simulink model "A1_cc_R2017b"  (R2020b)
settings: Solver=ode45  StartTime=0.0  StopTime=100  MaxStep=1e-3  RelTol=1e-3
values from neighbouring files (symbols this model uses):
  a = data(2)    [A1_10.m]    (also in problem6.m = 270)
  b = data(3)    [A1_10.m]    (also in problem6.m = 11000)
  g = 9.82    [A1_10.m]
  Ki = 0.0    (= 0)    [A1_10.m]
  Kp = 0.0    (= 0)    [A1_10.m]
settings Model: Creator=jofr  LastModifiedBy=jofr
settings DataIOCC: LimitDataPoints=on  SaveFormat=Array  SignalLoggingSaveFormat=ModelDataLogs  ReturnWorkspaceOutputs=off
settings OptimizationCC: BlockReduction=off  BooleanDataType=off  LifeSpan=inf
settings DebuggingCC: SaveWithParameterizedLinksMsg=none  UnderspecifiedInitializationDetection=Classic  MergeDetectMultiDrivingBlocksExec=none  SignalResolutionControl=TryResolveAllWithWarning  MultiTaskDSMMsg=warning  MultiTaskCondExecSysMsg=none  SFUnexpectedBacktrackingDiag=warning  SFNoUnconditionalDefaultTransitionDiag=warning  SFExecutionAtInitializationDiag=none  ArithmeticOperatorsInVariantConditions=warning
settings HardwareCC: ProdBitPerPointer=32  ProdBitPerSizeT=32  ProdBitPerPtrDiffT=32  ProdLargestAtomicFloat=None  ProdIntDivRoundTo=Undefined  ProdEndianess=Unspecified  ProdWordSize=32  ProdHWDeviceType=32-bit Generic  TargetUnknown=on
settings ModelReferenceCC: PropagateSignalLabelsOutOfModel=off
settings SFSimCC: SimUseLocalCustomCode=off  CustomCodeUndefinedFunction=UseInterfaceOnly
settings RTWCC: RTWUseLocalCustomCode=off
settings CodeAppCC: StateflowObjectComments=on
settings GRTTargetCC: TargetLangStandard=C89/C90 (ANSI)
settings ConfigComp: CovMetricSettings=dw  CovSaveCumulativeToWorkspaceVar=on  CovSaveSingleToWorkspaceVar=on  CovExternalEMLEnable=off

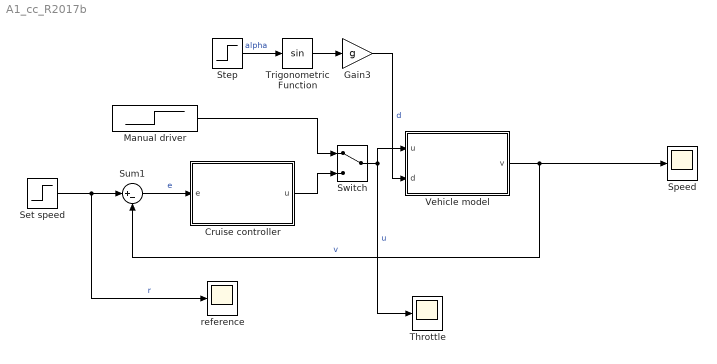
== system A1_cc_R2017b ==
  Cruise controller : Subsystem
  Gain3 : Gain  Gain=g
  Manual driver : Step  Before=25*a/b  After=30*a/b  SampleTime=0
  Set speed : Step  Before=25  After=30  SampleTime=0
  Speed : Scope
  Step : Step  Time=1000  After=0.1  SampleTime=0
  Sum1 : Sum  Inputs=|+-
  Switch : ManualSwitch
  Throttle : Scope
  Trigonometric Function : Trigonometry
  Vehicle model : Subsystem
  reference : Scope
  wires:
  Trigonometric Function/1 -> Gain3/1
  Step/1 -> Trigonometric Function/1  "alpha"
  Set speed/1 -> Sum1/1, reference/1  "r"
  Sum1/1 -> Cruise controller/1(e)  "e"
  Vehicle model/1(v) -> Sum1/2, Speed/1  "v"
  Gain3/1 -> Vehicle model/2(d)  "d"
  Switch/1 -> Throttle/1, Vehicle model/1(u)  "u"
  Cruise controller/1(u) -> Switch/2
  Manual driver/1 -> Switch/1

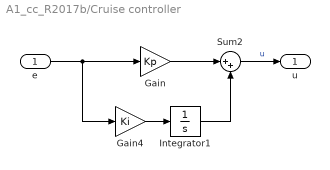
== system A1_cc_R2017b/Cruise controller ==
  e : Inport
  Gain : Gain  Gain=Kp
  Gain4 : Gain  Gain=Ki
  Integrator1 : Integrator  InitialCondition=a*25/b
  Sum2 : Sum  Inputs=|++
  u : Outport
  wires:
  Gain4/1 -> Integrator1/1
  Gain/1 -> Sum2/1
  Sum2/1 -> u/1  "u"
  Integrator1/1 -> Sum2/2
  e/1 -> Gain4/1, Gain/1

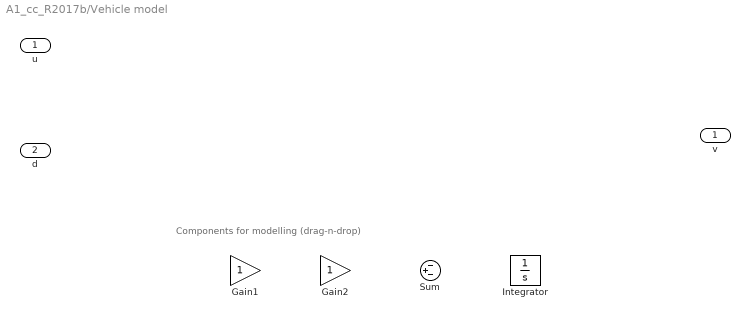
== system A1_cc_R2017b/Vehicle model ==
  note: Components for modelling (drag-n-drop)
  u : Inport
  d : Inport  Port=2
  Gain1 : Gain
  Gain2 : Gain
  Integrator : Integrator  InitialCondition=25
  Sum : Sum  Inputs=-+-
  v : Outport
